simulink model "MLC_LQR_benchmarking_Model_2020b_students"  (R2020b)
settings: Solver=FixedStepAuto  StartTime=0.0  StopTime=Tend  FixedStep=dt  RelTol=1e-3
undefined symbols (not defined in the file or in its folder): A, B, C, cost_threshold, D, InitCond, interpreter_kmlc, Q_MLC, R_MLC
libraries: simulink x1
settings Model: Creator=mario  LastModifiedBy=mario

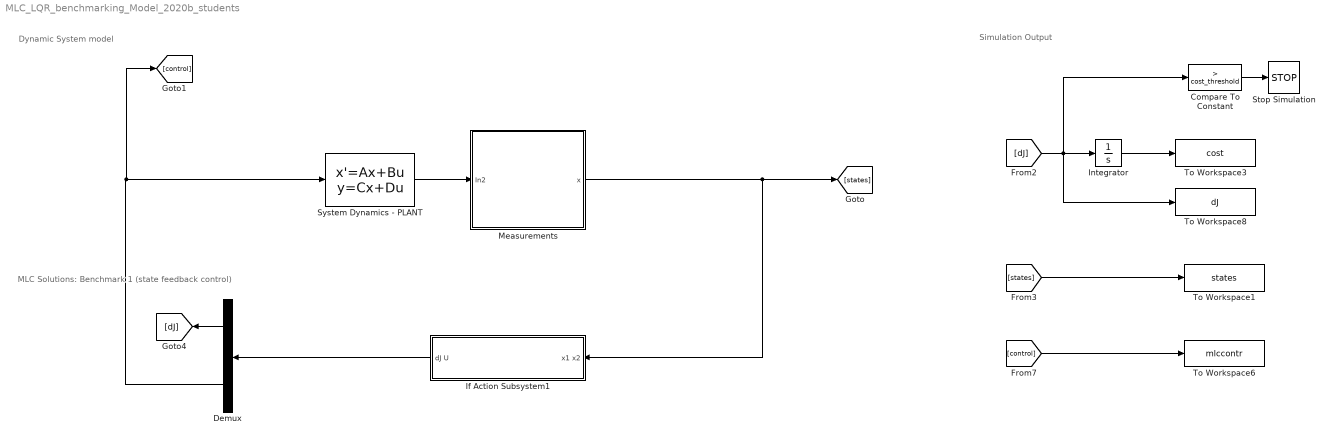
== system MLC_LQR_benchmarking_Model_2020b_students ==
  note: Dynamic System model
  note: MLC Solutions: Benchmark 1 (state feedback control)
  note: Simulation Output
  Compare To Constant : simulink/Logic and Bit Operations/Compare To Constant  relop=>  const=cost_threshold  OutDataTypeStr=boolean
  Demux : Demux  Outputs=[1 1]
  If Action Subsystem1 : Subsystem  TreatAsAtomicUnit=on
  Integrator : Integrator
  Measurements : Subsystem
  Stop Simulation : Stop
  System Dynamics - PLANT : StateSpace  A=A  B=B  C=C  D=D  InitialCondition=InitCond
  To Workspace1 : ToWorkspace  VariableName=states  SaveFormat=Timeseries  SampleTime=-1
  To Workspace3 : ToWorkspace  VariableName=cost  SaveFormat=Timeseries  SampleTime=-1
  To Workspace6 : ToWorkspace  VariableName=mlccontr  SaveFormat=Timeseries  SampleTime=-1
  To Workspace8 : ToWorkspace  VariableName=dJ  SaveFormat=Timeseries  SampleTime=-1
  wires:
  System Dynamics - PLANT/1 -> Measurements/1(In2)
  Compare To Constant/1 -> Stop Simulation/1
  Integrator/1 -> To Workspace3/1
  [dJ] -> Compare To Constant/1, Integrator/1, To Workspace8/1
  Measurements/1(x) -> [states], If Action Subsystem1/1(x1 x2)
  If Action Subsystem1/1(dJ U) -> Demux/1
  [states] -> To Workspace1/1
  [control] -> To Workspace6/1
  Demux/1 -> [dJ]
  Demux/2 -> [control], System Dynamics - PLANT/1

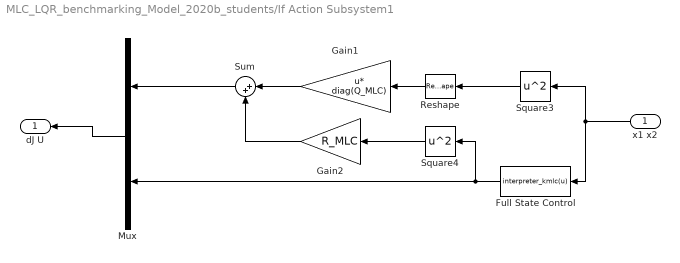
== system MLC_LQR_benchmarking_Model_2020b_students/If Action Subsystem1 ==
  x1 x2 : Inport
  Full State Control : MATLABFcn  MATLABFcn=interpreter_kmlc(u)  OutputDimensions=1  OutputSignalType=real
  Gain1 : Gain  Gain=diag(Q_MLC)  Multiplication=Matrix(u*K)
  Gain2 : Gain  Gain=R_MLC
  Mux : Mux  Inputs=[1 1]
  Reshape : Reshape  OutputDimensionality=Row vector (2-D)
  Square3 : Math  Operator=square  SaturateOnIntegerOverflow=on
  Square4 : Math  Operator=square  SaturateOnIntegerOverflow=on
  Sum : Sum  Inputs=|++
  dJ U : Outport
  wires:
  x1 x2/1 -> Full State Control/1, Square3/1
  Gain2/1 -> Sum/2
  Mux/1 -> dJ U/1
  Square3/1 -> Reshape/1
  Reshape/1 -> Gain1/1
  Square4/1 -> Gain2/1
  Gain1/1 -> Sum/1
  Full State Control/1 -> Square4/1, Mux/2
  Sum/1 -> Mux/1

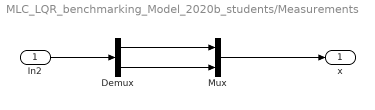
== system MLC_LQR_benchmarking_Model_2020b_students/Measurements ==
  In2 : Inport
  Demux : Demux  Outputs=2
  Mux : Mux  Inputs=2
  x : Outport
  wires:
  Demux/1 -> Mux/1
  Demux/2 -> Mux/2
  Mux/1 -> x/1
  In2/1 -> Demux/1
